simulink model "vdp2d"  (Simulink 3.00)
settings: Solver=ode45  SolverMode=SingleTasking  StartTime=0.0  StopTime=inf  RelTol=1e-3  AbsTol=1e-6
undefined symbols (not defined in the file or in its folder): sfunxyz
settings Model: ExternalInput=[]  SaveTime=off  SaveOutput=off  InitialState=[]  IntegerOverflowMsg=none  RTWOptions="-aEnforceIntegerDowncast=1 -aFoldNonRolledExpr=1 -aInlineInvariantSignals=1 -aInlineParameters=0 -aLocalBlockOutputs=1 -aRollThreshold=5 -aZeroInternalMemoryAtStartup=1 -aZeroExternalMemoryAtStartup=1 -aInitFltsAndDblsToZero=1 -aGenerateReport=0 -aGenCodeOnly=0 -aRTWVerbose=1 -aIncludeHyperlinkInReport=0 -aLaunchReport=0 -aForceParamTrailComments=0 -aGenerateComments=1 -aIgnoreCustomStorageClasses=1 -aIncHierarchyInIds=0 -aMaxRTWIdLen=31 -aShowEliminatedStatements=0 -aPrefixModelToSubsysFcnNames=1 -aIncDataTypeInIds=0 -aInsertBlockDesc=0 -aSimulinkBlockComments=1 -aInlinedPrmAccess=\"Literals\"  -aSuppressErrorStatus=0 -aModelReferenceCompliant=1 -aSupportNonInlinedSFcns=1 -aSupportContinuousTime=1 -aSupportComplex=1 -aSupportNonFinite=1 -aSupportAbsoluteTime=1 -aTargetFcnLib=\"ansi_tfl_tmw.mat\" -aMultiInstanceERTCode=0 -aLogVarNameModifier=\"rt_\" -aIsPILTarget=0 -aCombineOutputUpdateFcns=0 -aGenerateASAP2=0 -aGenerateSampleERTMain=0 -aGenerateFullHeader=1 -aUtilityFuncGeneration=\"Auto\" -aIncludeFileDelimiter=\"Auto\" -aIncludeMdlTerminateFcn=1 -aPurelyIntegerCode=0 -aERTCustomFileBanners=0 -aRTWCAPIStates=0 -aRTWCAPIParams=0 -aRTWCAPISignals=0 -aMatFileLogging=1 -aGenFloatMathFcnCalls=\"ANSI_C\" -aExtModeMexFile=\"ext_comm\" -aExtModeTransport=0 -aExtModeStaticAllocSize=1000000 -aExtModeTesting=0 -aExtModeStaticAlloc=0 -aExtMode=0  -aInitFltsAndDblsToZero=1 -aInitFltsAndDblsToZero=1"  Creator=The MathWorks Inc.  LastModifiedBy=campa

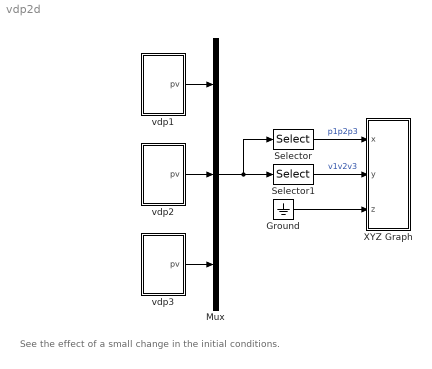
== system vdp2d ==
  note: See the effect of a small change in the initial conditions.
  Ground : Ground
  Mux : Mux  Inputs=[2 2 2]
  Selector : Selector  Elements=[1 3 5]  InputPortWidth=6
  Selector1 : Selector  Elements=[2 4 6]  InputPortWidth=6
  XYZ Graph : Subsystem  LoadFcn=sfunxyz([],[],[],'LoadBlock')  StartFcn=sfunxyz([],[],[],'Start')  StopFcn=sfunxyz([],[],[],'Stop')  mask(XYZ multiscope){np=3, xlim=[-3 3], ylim=[-3 3], zlim=[0 1], cp=[0 0 1], gd=on, st=0.01}
      mask prompts: np "Number of lines"; xlim "[xmin xmax]"; ylim "[ymin ymax]"; zlim "[zmin zmax]"; cp "Camera position (use [0 0 1] for 2D XY view)"; gd "Grid"; st "Sample time:"
      mask help:
      | Multidimensional XYZ scope using MATLAB graph window.
      |    X,Y,Z coordinates are respectively the first,second, and third input.
      |    Enter the number of lines, the XYZ ranges, the camera position,
      |    and the sampling time, as mask parameters.
      settings: CopyFcn=sfunxyz([],[],[],'CopyBlock')  DeleteFcn=sfunxyz([],[],[],'DeleteBlock')  NameChangeFcn=sfunxyz([],[],[],'NameChange')
      mask Help:
      | This block can be used to explore limit cycles.
      |    Look at the m-file sfunxyz.m to see how it works.
      mask Display: plot([.05 .95 .95 .05 .05],[.45 .45 .95 .95 .45], 0.5+cos(0:0.1:2*pi)*0.3,0.7+sin(0:0.1:2*pi)*0.2)
  vdp1 : Subsystem  mask(Van Der Pol System){mu=1, p0=0.5, v0=0}
      mask prompts: p0 "Initial position (x1)"; v0 "Initial velocity (x2)"
      mask help:
      | This autonomous system represents the van der pol equation:
      | pdot=v; vdot=mu*v*(1-p^2)*-p;
      | Parameters and initial state can be selected from the mask.
      mask Help:
      | This autonomous system represents the van der pol equation:
      | Parameters and initial state can be selected from the mask.
      | <p>
      | The system equations are:
      | pdot=v;
      | vdot=mu*v*(1-p^2)*-p;
  vdp2 : Subsystem  mask(Van Der Pol System){mu=1, p0=1, v0=0}
      mask prompts: p0 "Initial position (x1)"; v0 "Initial velocity (x2)"
      mask help:
      | This autonomous system represents the van der pol equation:
      | pdot=v; vdot=mu*v*(1-p^2)*-p;
      | Parameters and initial state can be selected from the mask.
      mask Help:
      | This autonomous system represents the van der pol equation:
      | Parameters and initial state can be selected from the mask.
      | <p>
      | The system equations are:
      | pdot=v;
      | vdot=mu*v*(1-p^2)*-p;
  vdp3 : Subsystem  mask(Van Der Pol System){mu=1, p0=1.5, v0=0}
      mask prompts: p0 "Initial position (x1)"; v0 "Initial velocity (x2)"
      mask help:
      | This autonomous system represents the van der pol equation:
      | pdot=v; vdot=mu*v*(1-p^2)*-p;
      | Parameters and initial state can be selected from the mask.
      mask Help:
      | This autonomous system represents the van der pol equation:
      | Parameters and initial state can be selected from the mask.
      | <p>
      | The system equations are:
      | pdot=v;
      | vdot=mu*v*(1-p^2)*-p;
  wires:
  vdp1/1(pv) -> Mux/1
  Mux/1 -> Selector/1, Selector1/1
  Selector/1 -> XYZ Graph/1(x)  "p1p2p3"
  Selector1/1 -> XYZ Graph/2(y)  "v1v2v3"
  Ground/1 -> XYZ Graph/3(z)
  vdp2/1(pv) -> Mux/2
  vdp3/1(pv) -> Mux/3

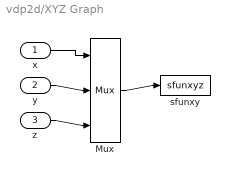
== system vdp2d/XYZ Graph ==
  x : Inport  Port=1  PortWidth=-1  SampleTime=-1  DataType=auto
      settings: SignalType=auto
  y : Inport  Port=2  PortWidth=-1  SampleTime=-1  DataType=auto
      settings: SignalType=auto
  z : Inport  Port=3  PortWidth=-1  SampleTime=-1  DataType=auto
      settings: SignalType=auto
  Mux : Mux  Inputs=[np np np]
      settings: DisplayOption=none
  sfunxy : S-Function  FunctionName=sfunxyz  Parameters=[xlim ylim zlim],st,np,cp,gd  PortCounts=[]  SFunctionModules=''
  wires:
  Mux/1 -> sfunxy/1
  x/1 -> Mux/1
  y/1 -> Mux/2
  z/1 -> Mux/3

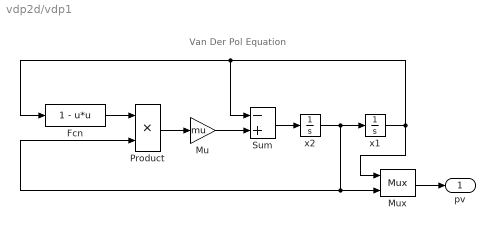
== system vdp2d/vdp1 ==
  note: Van Der Pol Equation
  Fcn : Fcn  Expr=1 - u*u
  Mu : Gain  Gain=mu  SaturateOnIntegerOverflow=on
  Mux : Mux  Inputs=2
      settings: DisplayOption=none
  Product : Product  Inputs=2  SaturateOnIntegerOverflow=on
  Sum : Sum  Inputs=-+  SaturateOnIntegerOverflow=on
  x1 : Integrator  ExternalReset=none  InitialConditionSource=internal  InitialCondition=p0  LimitOutput=off  UpperSaturationLimit=inf  LowerSaturationLimit=-inf  ShowSaturationPort=off  ShowStatePort=off  AbsoluteTolerance=auto
  x2 : Integrator  ExternalReset=none  InitialConditionSource=internal  InitialCondition=v0  LimitOutput=off  UpperSaturationLimit=inf  LowerSaturationLimit=-inf  ShowSaturationPort=off  ShowStatePort=off  AbsoluteTolerance=auto
  pv : Outport  Port=1
  wires:
  Sum/1 -> x2/1
  x2/1 -> x1/1, Mux/2, Product/2
  x1/1 -> Mux/1, Fcn/1, Sum/1
  Mux/1 -> pv/1
  Product/1 -> Mu/1
  Mu/1 -> Sum/2
  Fcn/1 -> Product/1

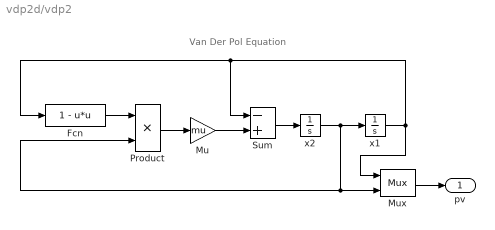
== system vdp2d/vdp2 ==
  note: Van Der Pol Equation
  Fcn : Fcn  Expr=1 - u*u
  Mu : Gain  Gain=mu  SaturateOnIntegerOverflow=on
  Mux : Mux  Inputs=2
      settings: DisplayOption=none
  Product : Product  Inputs=2  SaturateOnIntegerOverflow=on
  Sum : Sum  Inputs=-+  SaturateOnIntegerOverflow=on
  x1 : Integrator  ExternalReset=none  InitialConditionSource=internal  InitialCondition=p0  LimitOutput=off  UpperSaturationLimit=inf  LowerSaturationLimit=-inf  ShowSaturationPort=off  ShowStatePort=off  AbsoluteTolerance=auto
  x2 : Integrator  ExternalReset=none  InitialConditionSource=internal  InitialCondition=v0  LimitOutput=off  UpperSaturationLimit=inf  LowerSaturationLimit=-inf  ShowSaturationPort=off  ShowStatePort=off  AbsoluteTolerance=auto
  pv : Outport  Port=1
  wires:
  Fcn/1 -> Product/1
  Mu/1 -> Sum/2
  Product/1 -> Mu/1
  Mux/1 -> pv/1
  x1/1 -> Sum/1, Fcn/1, Mux/1
  x2/1 -> Product/2, Mux/2, x1/1
  Sum/1 -> x2/1

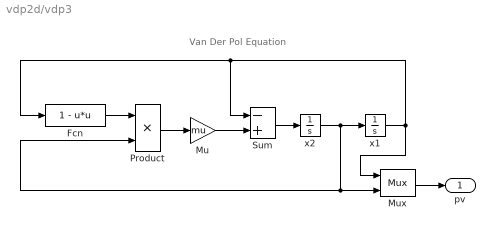
== system vdp2d/vdp3 ==
  note: Van Der Pol Equation
  Fcn : Fcn  Expr=1 - u*u
  Mu : Gain  Gain=mu  SaturateOnIntegerOverflow=on
  Mux : Mux  Inputs=2
      settings: DisplayOption=none
  Product : Product  Inputs=2  SaturateOnIntegerOverflow=on
  Sum : Sum  Inputs=-+  SaturateOnIntegerOverflow=on
  x1 : Integrator  ExternalReset=none  InitialConditionSource=internal  InitialCondition=p0  LimitOutput=off  UpperSaturationLimit=inf  LowerSaturationLimit=-inf  ShowSaturationPort=off  ShowStatePort=off  AbsoluteTolerance=auto
  x2 : Integrator  ExternalReset=none  InitialConditionSource=internal  InitialCondition=v0  LimitOutput=off  UpperSaturationLimit=inf  LowerSaturationLimit=-inf  ShowSaturationPort=off  ShowStatePort=off  AbsoluteTolerance=auto
  pv : Outport  Port=1
  wires:
  Sum/1 -> x2/1
  x2/1 -> x1/1, Mux/2, Product/2
  x1/1 -> Mux/1, Fcn/1, Sum/1
  Mux/1 -> pv/1
  Product/1 -> Mu/1
  Mu/1 -> Sum/2
  Fcn/1 -> Product/1
